simulink model "ClosedLoop_CqCscCi"  (R2023b)
settings: Solver=VariableStepAuto  StartTime=0.0  StopTime=10.0  RelTol=1e-6
libraries: cstblocks x5
settings Model: Creator=bolee  LastModifiedBy=bolee

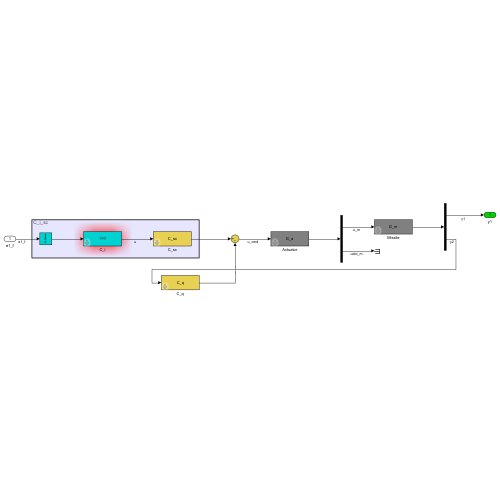
[thumbnail: Simulink's stored preview of the top-level diagram]
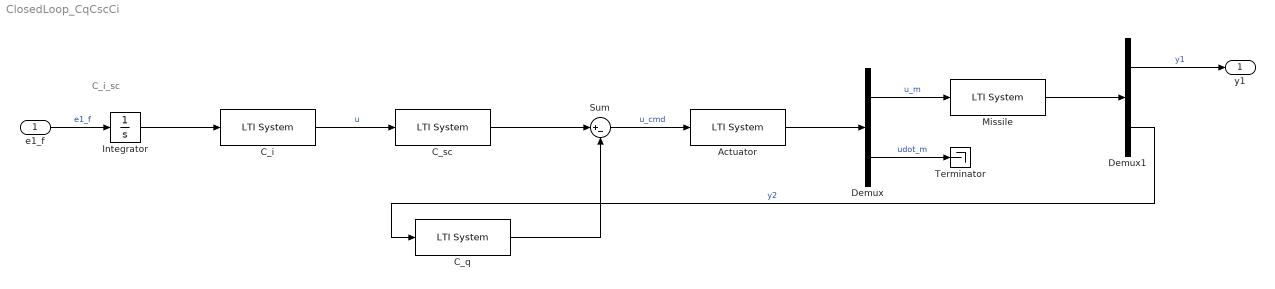
== system ClosedLoop_CqCscCi ==
  note: C_i_sc
  e1_f : Inport
  Actuator : cstblocks/LTI System  sys=G_a  IC=[]  PadeOrder=0
  C_i : cstblocks/LTI System  sys=C_i  IC=[]  PadeOrder=0
  C_q : cstblocks/LTI System  sys=C_q  IC=[]  PadeOrder=0
  C_sc : cstblocks/LTI System  sys=C_sc  IC=[]  PadeOrder=0
  Demux : Demux  Outputs=2
  Demux1 : Demux  Outputs=2
  Integrator : Integrator
  Missile : cstblocks/LTI System  sys=G_m  IC=[]  PadeOrder=0
  Sum : Sum  Inputs=|+-
  Terminator : Terminator
  y1 : Outport
  wires:
  Actuator/1 -> Demux/1
  Sum/1 -> Actuator/1  "u_cmd"
  Demux/1 -> Missile/1  "u_m"
  Demux/2 -> Terminator/1  "udot_m"
  Missile/1 -> Demux1/1
  Demux1/1 -> y1/1  "y1"
  C_q/1 -> Sum/2
  Demux1/2 -> C_q/1  "y2"
  e1_f/1 -> Integrator/1  "e1_f"
  C_sc/1 -> Sum/1
  Integrator/1 -> C_i/1
  C_i/1 -> C_sc/1  "u"
